simulink model "sf_carcctrl_xpc"  (Simulink 6.0)
settings: Solver=ode4  SolverMode=SingleTasking  StartTime=0.0  StopTime=inf  FixedStep=0.001  RelTol=1e-3  AbsTol=1e-6
PreLoadFcn:
  | load sf_cardat
undefined symbols (not defined in the file or in its folder): converter_data, downtab, emap, Iei, uptab
libraries: xpclib x3, simulink_extras x1
settings Model: CovMetricSettings=d  Creator=nikita  LastModifiedBy=ekbas  ExtModeTrigMode=oneshot  ExtModeArmWhenConnect=off  BufferReuse=off
settings DataIOCC: LimitDataPoints=off  SaveOutput=off  SaveTime=off  SignalLoggingName=sigsOut
settings OptimizationCC: BlockReduction=off  BooleanDataType=off  InlineInvariantSignals=off  OptimizeBlockIOStorage=off  BufferReuse=off  EnforceIntegerDowncast=off  FoldNonRolledExpr=off  LocalBlockOutputs=off
settings DebuggingCC: CheckExecutionContextPreStartOutputMsg=on  CheckExecutionContextRuntimeOutputMsg=on  SolverPrmCheckMsg=none  IntegerOverflowMsg=none
settings RTWCC: SystemTargetFile=xpctarget.tlc  TemplateMakefile=xpc_default_tmf  ProcessScript=xpctarget_make_rtw_hook
settings xpcTargetCC: TargetFcnLib=ansi_tfl_tmw.mat  GenFloatMathFcnCalls=ANSI_C  ModelReferenceCompliant=off  LifeSpan=inf
settings SFSimCC: SFSimApplyToAllLibs=on  SFSimBuildMode=Incremental

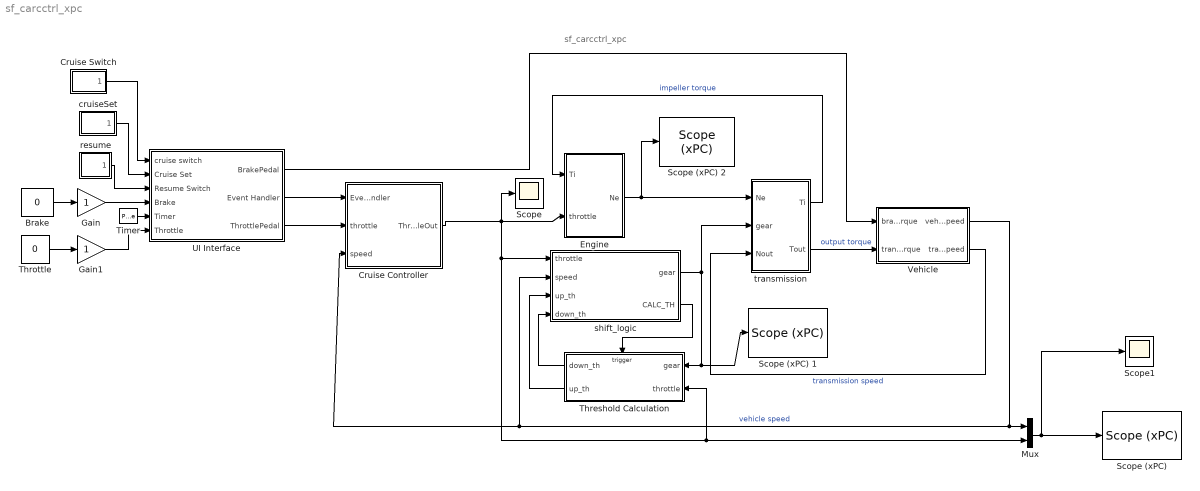
== system sf_carcctrl_xpc ==
  note: sf_carcctrl_xpc
  Brake : Constant  Value=0
  Cruise Controller : Subsystem  PropExecContextAcrossSSBoundary=on
  Cruise Switch : Subsystem  PropExecContextAcrossSSBoundary=on  mask(Manual Switch){sw=1, action=0}
      mask prompts: sw "Current setting:"
      mask help: Output toggles between two inputs by double-clicking on the block.
      mask init:
      | [x,y]=manevent;
      settings: OpenFcn=set_param(gcbh,'action','1');
      mask Help: This block implements a manual switch.
      mask Display: plot(x,y);
  Engine : Subsystem  PropExecContextAcrossSSBoundary=on
  Gain : Gain  SaturateOnIntegerOverflow=on
  Gain1 : Gain  SaturateOnIntegerOverflow=on
  Mux : Mux  Inputs=2
  Scope : Scope
      settings: TimeRange=10  YMin=-1  YMax=1
  "Scope (xPC) " : xpclib/Misc./Scope (xPC)   scopeno=1  scopetype=Target  autostart=on  viewmode=Graphical rolling  formatstr='%15.6f'  grid=on  ylimits=[0,160]  nosamples=1000  noprepostsamples=0  interleave=50  triggermode=FreeRun  triggersignal=1  triggerlevel=0.0  triggerslope=Either  triggerscope=1  triggersample=0  filename=data.dat  mode=Lazy  writesize=512  autorestart=off
  Scope (xPC) 1 : xpclib/Misc./Scope (xPC)   scopeno=3  scopetype=Target  autostart=on  viewmode=Numerical  formatstr='%15.6f'  grid=on  ylimits=[0,180]  nosamples=50  noprepostsamples=0  interleave=1  triggermode=FreeRun  triggersignal=1  triggerlevel=0.0  triggerslope=Either  triggerscope=1  triggersample=0  filename=data.dat  mode=Lazy  writesize=512  autorestart=off
  Scope (xPC) 2 : xpclib/Misc./Scope (xPC)   scopeno=2  scopetype=Target  autostart=on  viewmode=Graphical rolling  formatstr='%15.6f'  grid=on  ylimits=[0,6000]  nosamples=1000  noprepostsamples=0  interleave=50  triggermode=FreeRun  triggersignal=1  triggerlevel=0.0  triggerslope=Either  triggerscope=1  triggersample=0  filename=data.dat  mode=Lazy  writesize=512  autorestart=off
  Scope1 : Scope
      settings: TimeRange=10  YMin=0  YMax=5.5  SaveName=ScopeData2
  Threshold Calculation : Subsystem  Orientation=left  TreatAsAtomicUnit=on  PropExecContextAcrossSSBoundary=on
  Throttle : Constant  Value=0
  Timer : DiscretePulseGenerator  PulseType=Time based  Period=0.05  PulseWidth=50
  UI Interface : Subsystem  PropExecContextAcrossSSBoundary=on
  Vehicle : Subsystem  PropExecContextAcrossSSBoundary=on  mask(vehicle model){@1=vehicledata(1), @2=vehicledata(2), @3=vehicledata(3), @4=vehicledata(4), @5=vehicledata(5), @6=vehicledata(6)/vehicledata(4)*vehicledata(1)}
      mask prompts: @1 "final drive ratio"; @2 "drag friction at wheels"; @3 "aerodynamic drag"; @4 "wheel radius"; @5 "vehicle inertia"; @6 "initial transmission output speed"
      mask help: vehicle dynamics: torque input from trans., outputs are input speed (transmission output) and vehicle speed
      mask init:
      | Rfd = @1; rload0 = @2; rload2 = @3; Rw = @4; Iv = @5; N20 = @6;
      mask Display: plot([cos(pi*[0:5:360]/180) + 6], [sin(pi*[0:5:360]/180) + 1.5],[cos(pi*[0:5:360]/180) + 1], [sin(pi*[0:5:360]/180) + 4], [10 7.5 6.75], [3.5 1 1.5], [10 9.75 7.5 6.25 3 1.5 4 5 7.5], [3.5 4.75 5.5 7 8 7 6 4 5.5], [6.5 4], [7 6], [5.25 2], [2 4], [7.5 1 0], [2.5 6 6.5], [7.5 7.25 9.75], [1 2.25 4.75], [2.75 2 0 0 0.25], [7.5 8 6.5 5.25 5], [1.5 0.5], [6.75 6.25])
  cruiseSet : Subsystem  PropExecContextAcrossSSBoundary=on  mask(Manual Switch){sw=1, action=0}
      mask prompts: sw "Current setting:"
      mask help: Output toggles between two inputs by double-clicking on the block.
      mask init:
      | [x,y]=manevent;
      settings: OpenFcn=set_param(gcbh,'action','1');
      mask Help: This block implements a manual switch.
      mask Display: plot(x,y);
  resume : Subsystem  PropExecContextAcrossSSBoundary=on  mask(Manual Switch){sw=0, action=0}
      mask prompts: sw "Current setting:"
      mask help: Output toggles between two inputs by double-clicking on the block.
      mask init:
      | [x,y]=manevent;
      settings: OpenFcn=set_param(gcbh,'action','1');
      mask Help: This block implements a manual switch.
      mask Display: plot(x,y);
  shift_logic : Stateflow chart  PropExecContextAcrossSSBoundary=on
  transmission : Subsystem  PropExecContextAcrossSSBoundary=on
  wires:
  transmission/1(Ti) -> Engine/1(Ti)  "impeller torque"
  Engine/1(Ne) -> transmission/1(Ne), Scope (xPC) 2/1
  transmission/2(Tout) -> Vehicle/2(transmission output torque)  "output torque"
  Vehicle/2(transmission output speed) -> transmission/3(Nout)  "transmission speed"
  Threshold Calculation/1(down_th) -> shift_logic/4(down_th)
  Threshold Calculation/2(up_th) -> shift_logic/3(up_th)
  shift_logic/1(gear) -> transmission/2(gear), Threshold Calculation/1(gear), Scope (xPC) 1/1
  shift_logic/2(CALC_TH) -> Threshold Calculation/Trigger
  Vehicle/1(vehicle speed) -> Mux/1, shift_logic/2(speed), Cruise Controller/3(speed)  "vehicle speed"
  Mux/1 -> "Scope (xPC) "/1, Scope1/1
  Cruise Controller/1(ThrottleOut) -> shift_logic/1(throttle), Mux/2, Threshold Calculation/2(throttle), Engine/2(throttle), Scope/1
  Throttle/1 -> Gain1/1
  Timer/1 -> UI Interface/5(Timer)
  cruiseSet/1(Output) -> UI Interface/2(Cruise Set)
  resume/1(Output) -> UI Interface/3(Resume Switch)
  Cruise Switch/1(Output) -> UI Interface/1(cruise switch)
  Brake/1 -> Gain/1
  UI Interface/2(Event Handler) -> Cruise Controller/1(Event Handler)
  UI Interface/3(ThrottlePedal) -> Cruise Controller/2(throttle)
  UI Interface/1(BrakePedal) -> Vehicle/1(brake torque)
  Gain/1 -> UI Interface/4(Brake)
  Gain1/1 -> UI Interface/6(Throttle)

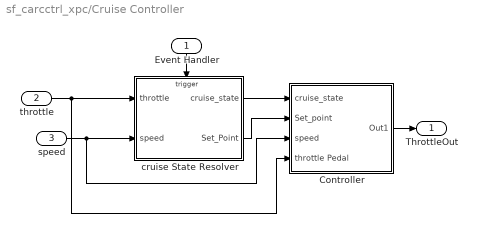
== system sf_carcctrl_xpc/Cruise Controller ==
  Event Handler : Inport  Orientation=down  LatchInput=off
  throttle : Inport  Port=2  LatchInput=off
  speed : Inport  Port=3  LatchInput=off
  Controller : Subsystem  PropExecContextAcrossSSBoundary=on
  cruise State Resolver : Stateflow chart  TreatAsAtomicUnit=on  PropExecContextAcrossSSBoundary=on
  ThrottleOut : Outport
  wires:
  Controller/1(Out1) -> ThrottleOut/1
  Event Handler/1 -> cruise State Resolver/Trigger
  speed/1 -> Controller/3(speed), cruise State Resolver/2(speed)
  throttle/1 -> Controller/4(throttle Pedal), cruise State Resolver/1(throttle)
  cruise State Resolver/2(Set_Point) -> Controller/2(Set_point)
  cruise State Resolver/1(cruise_state) -> Controller/1(cruise_state)

== system sf_carcctrl_xpc/Cruise Switch ==
  Constant : Constant
  Output : Outport
  wires:
  Constant/1 -> Output/1

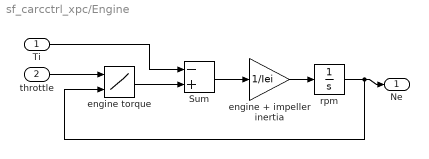
== system sf_carcctrl_xpc/Engine ==
  Ti : Inport  LatchInput=off
  throttle : Inport  Port=2  LatchInput=off
  Sum : Sum  Inputs=-+  SaturateOnIntegerOverflow=on  InputSameDT=on
  engine torque : Lookup2D  DialogController=Simulink.DDGSource  RowIndex=thvec  ColumnIndex=nevec  OutputValues=emap  SaturateOnIntegerOverflow=on  InputSameDT=on
  engine + impeller inertia : Gain  Gain=1/Iei  SaturateOnIntegerOverflow=on
  rpm : Integrator  InitialCondition=1000  LimitOutput=on  UpperSaturationLimit=6000  LowerSaturationLimit=600
  Ne : Outport  InitialOutput=0
  wires:
  Ti/1 -> Sum/1
  throttle/1 -> engine torque/1
  rpm/1 -> engine torque/2, Ne/1
  Sum/1 -> engine + impeller inertia/1
  engine + impeller inertia/1 -> rpm/1
  engine torque/1 -> Sum/2

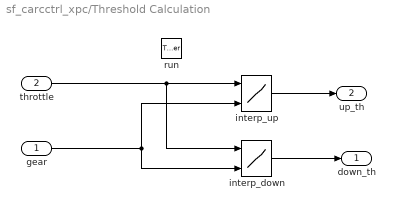
== system sf_carcctrl_xpc/Threshold Calculation ==
  gear : Inport  LatchInput=off
  throttle : Inport  Port=2  LatchInput=off
  run : TriggerPort  TriggerType=function-call  StatesWhenEnabling=reset
  interp_down : Lookup2D  DialogController=Simulink.DDGSource  RowIndex=downth  ColumnIndex=[1:4]  OutputValues=downtab  SaturateOnIntegerOverflow=on  InputSameDT=on
  interp_up : Lookup2D  DialogController=Simulink.DDGSource  RowIndex=upth  ColumnIndex=[1:4]  OutputValues=uptab  SaturateOnIntegerOverflow=on  InputSameDT=on
  down_th : Outport
  up_th : Outport  Port=2
  wires:
  interp_up/1 -> up_th/1
  interp_down/1 -> down_th/1
  throttle/1 -> interp_up/1, interp_down/1
  gear/1 -> interp_up/2, interp_down/2

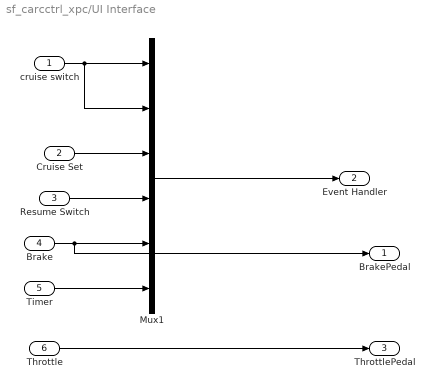
== system sf_carcctrl_xpc/UI Interface ==
  cruise switch : Inport  LatchInput=off
  Cruise Set : Inport  Port=2  LatchInput=off
  Resume Switch : Inport  Port=3  LatchInput=off
  Brake : Inport  Port=4  LatchInput=off
  Timer : Inport  Port=5  LatchInput=off
  Throttle : Inport  Port=6  LatchInput=off
  Mux1 : Mux  Inputs=6
  BrakePedal : Outport
  Event Handler : Outport  Port=2
  ThrottlePedal : Outport  Port=3
  wires:
  Throttle/1 -> ThrottlePedal/1
  Timer/1 -> Mux1/6
  Resume Switch/1 -> Mux1/4
  Cruise Set/1 -> Mux1/3
  cruise switch/1 -> Mux1/1, Mux1/2
  Mux1/1 -> Event Handler/1
  Brake/1 -> BrakePedal/1, Mux1/5

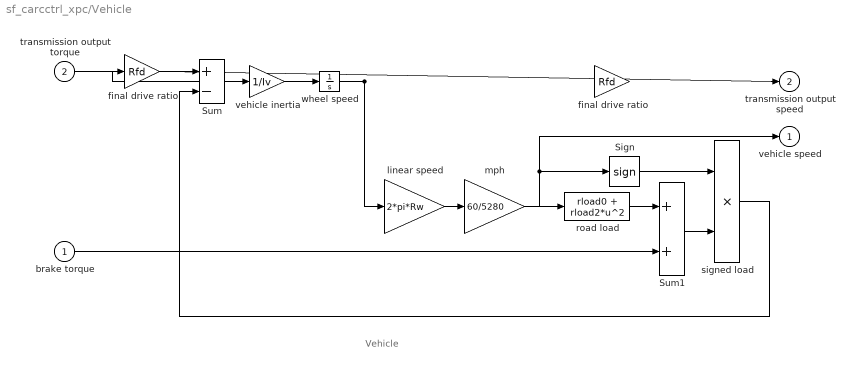
== system sf_carcctrl_xpc/Vehicle ==
  note: Vehicle
  brake torque : Inport  LatchInput=off
  transmission output torque : Inport  Port=2  LatchInput=off
  Sign : Signum
  Sum : Sum  Inputs=+-  SaturateOnIntegerOverflow=on  InputSameDT=on
  Sum1 : Sum  SaturateOnIntegerOverflow=on  InputSameDT=on
  final drive ratio : Gain  Gain=Rfd  SaturateOnIntegerOverflow=on
  final drive ratio : Gain  Gain=Rfd  SaturateOnIntegerOverflow=on
  linear speed : Gain  Gain=2*pi*Rw  SaturateOnIntegerOverflow=on
  mph : Gain  Gain=60/5280  SaturateOnIntegerOverflow=on
  road load : Fcn  Expr=rload0 + rload2*u^2
  signed load : Product  SaturateOnIntegerOverflow=on  InputSameDT=on
  vehicle inertia : Gain  Gain=1/Iv  SaturateOnIntegerOverflow=on
  wheel speed : Integrator  InitialCondition=N20/Rfd
  vehicle speed : Outport  InitialOutput=0
  transmission output speed : Outport  Port=2  InitialOutput=0
  wires:
  final drive ratio/1 -> transmission output speed/1
  brake torque/1 -> Sum1/2
  Sum1/1 -> signed load/2
  road load/1 -> Sum1/1
  Sign/1 -> signed load/1
  signed load/1 -> Sum/2
  transmission output torque/1 -> final drive ratio/1
  vehicle inertia/1 -> wheel speed/1
  Sum/1 -> vehicle inertia/1
  mph/1 -> vehicle speed/1, Sign/1, road load/1
  linear speed/1 -> mph/1
  wheel speed/1 -> linear speed/1, final drive ratio/1
  final drive ratio/1 -> Sum/1

== system sf_carcctrl_xpc/cruiseSet ==
  Constant : Constant
  Output : Outport
  wires:
  Constant/1 -> Output/1

== system sf_carcctrl_xpc/resume ==
  Constant : Constant  Value=0
  Output : Outport
  wires:
  Constant/1 -> Output/1

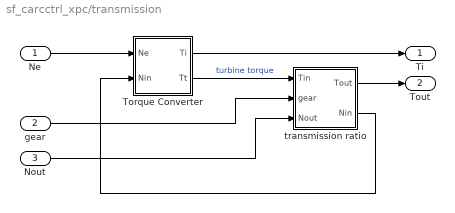
== system sf_carcctrl_xpc/transmission ==
  Ne : Inport  LatchInput=off
  gear : Inport  Port=2  LatchInput=off
  Nout : Inport  Port=3  LatchInput=off
  Torque Converter : Subsystem  PropExecContextAcrossSSBoundary=on  mask(torque converter){speedratio=converter_data(:,1), Kfactor=converter_data(:,2), Torkratio=converter_data(:,3)}
      mask prompts: speedratio "speed ratio"; Kfactor "K factor"; Torkratio "torque ratio"
      mask help: torque converter
      mask Help: Torque converter input and output torques are computed as a function of the input and output speeds
      mask Display: plot([cos([90:10:450]*pi/180),.63*cos([90:10:450]*pi/180),.63*cos([90:10:240]*pi/180),cos([240:10:300]*pi/180),.63*cos([300]*pi/180)],[sin([90:10:450]*pi/180),.63*sin([90:10:450]*pi/180)+.1,.63*sin([90:10:240]*pi/180)+.1,sin([240:10:300]*pi/180),.63*sin([300]*pi/180)+.1])
  transmission ratio : Subsystem  PropExecContextAcrossSSBoundary=on
  Ti : Outport  InitialOutput=0
  Tout : Outport  Port=2  InitialOutput=0
  wires:
  transmission ratio/1(Tout) -> Tout/1
  Torque Converter/1(Ti) -> Ti/1
  Nout/1 -> transmission ratio/3(Nout)
  gear/1 -> transmission ratio/2(gear)
  Ne/1 -> Torque Converter/1(Ne)
  transmission ratio/2(Nin) -> Torque Converter/2(Nin)
  Torque Converter/2(Tt) -> transmission ratio/1(Tin)  "turbine torque"

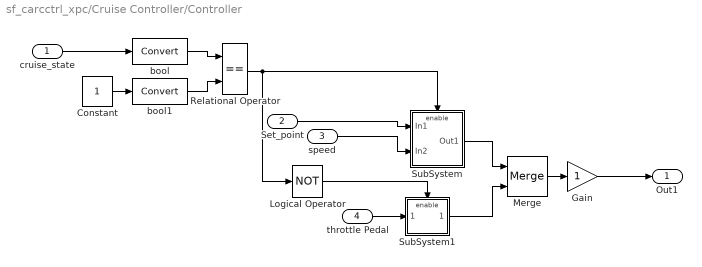
== system sf_carcctrl_xpc/Cruise Controller/Controller ==
  cruise_state : Inport  LatchInput=off
  Set_point : Inport  Port=2  LatchInput=off
  speed : Inport  Port=3  LatchInput=off
  throttle Pedal : Inport  Port=4  LatchInput=off
  Constant : Constant
  Gain : Gain  SaturateOnIntegerOverflow=on
  Logical Operator : Logic  Operator=NOT
  Merge : Merge
  Relational Operator : RelationalOperator  Operator===  InputSameDT=on
  SubSystem : Subsystem  TreatAsAtomicUnit=on  PropExecContextAcrossSSBoundary=on
  SubSystem1 : Subsystem  TreatAsAtomicUnit=on  PropExecContextAcrossSSBoundary=on
  bool : DataTypeConversion  OutDataTypeMode=boolean  SaturateOnIntegerOverflow=on  RndMeth=Zero
  bool1 : DataTypeConversion  OutDataTypeMode=boolean  SaturateOnIntegerOverflow=on  RndMeth=Zero
  Out1 : Outport  InitialOutput=0
  wires:
  Gain/1 -> Out1/1
  Merge/1 -> Gain/1
  SubSystem1/1(Out1) -> Merge/2
  SubSystem/1(Out1) -> Merge/1
  Logical Operator/1 -> SubSystem1/Enable
  Relational Operator/1 -> Logical Operator/1, SubSystem/Enable
  bool1/1 -> Relational Operator/2
  bool/1 -> Relational Operator/1
  throttle Pedal/1 -> SubSystem1/1(In1)
  Set_point/1 -> SubSystem/1(In1)
  Constant/1 -> bool1/1
  cruise_state/1 -> bool/1
  speed/1 -> SubSystem/2(In2)

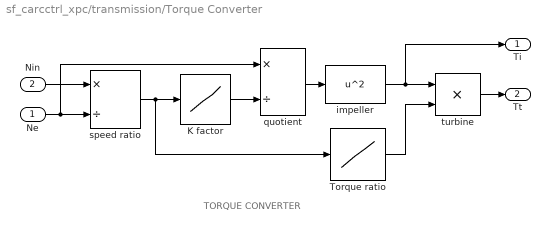
== system sf_carcctrl_xpc/transmission/Torque Converter ==
  note: TORQUE CONVERTER
  Ne : Inport  LatchInput=off
  Nin : Inport  Port=2  LatchInput=off
  K factor : Lookup  DialogController=Simulink.DDGSource  InputValues=speedratio  OutputValues=Kfactor  SaturateOnIntegerOverflow=on
  Torque ratio : Lookup  DialogController=Simulink.DDGSource  InputValues=speedratio  OutputValues=Torkratio  SaturateOnIntegerOverflow=on
  impeller : Fcn  Expr=u^2
  quotient : Product  Inputs=*/  SaturateOnIntegerOverflow=on  InputSameDT=on
  speed ratio : Product  Inputs=*/  SaturateOnIntegerOverflow=on  InputSameDT=on
  turbine : Product  SaturateOnIntegerOverflow=on  InputSameDT=on
  Ti : Outport  InitialOutput=0
  Tt : Outport  Port=2  InitialOutput=0
  wires:
  Torque ratio/1 -> turbine/2
  quotient/1 -> impeller/1
  K factor/1 -> quotient/2
  speed ratio/1 -> Torque ratio/1, K factor/1
  impeller/1 -> turbine/1, Ti/1
  turbine/1 -> Tt/1
  Ne/1 -> speed ratio/2, quotient/1
  Nin/1 -> speed ratio/1

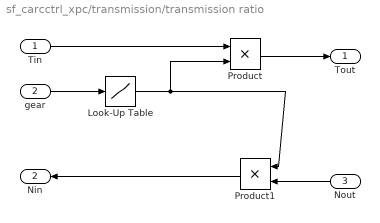
== system sf_carcctrl_xpc/transmission/transmission ratio ==
  Tin : Inport  LatchInput=off
  gear : Inport  Port=2  LatchInput=off
  Nout : Inport  Orientation=left  Port=3  LatchInput=off
  Look-Up Table : Lookup  DialogController=Simulink.DDGSource  InputValues=[1 2 3 4]  OutputValues=[2.393 1.450 1.000 0.677]  SaturateOnIntegerOverflow=on
  Product : Product  SaturateOnIntegerOverflow=on  InputSameDT=on
  Product1 : Product  Orientation=left  SaturateOnIntegerOverflow=on  InputSameDT=on
  Tout : Outport  InitialOutput=0
  Nin : Outport  Orientation=left  Port=2  InitialOutput=0
  wires:
  Look-Up Table/1 -> Product1/1, Product/2
  Nout/1 -> Product1/2
  Product1/1 -> Nin/1
  Product/1 -> Tout/1
  Tin/1 -> Product/1
  gear/1 -> Look-Up Table/1

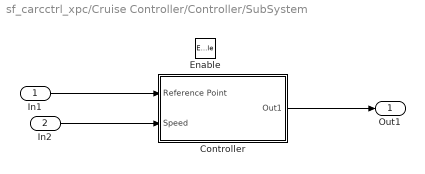
== system sf_carcctrl_xpc/Cruise Controller/Controller/SubSystem ==
  In1 : Inport  LatchInput=off
  In2 : Inport  Port=2  LatchInput=off
  Enable : EnablePort
  Controller : Subsystem  PropExecContextAcrossSSBoundary=on
  Out1 : Outport
  wires:
  In1/1 -> Controller/1(Reference Point)
  In2/1 -> Controller/2(Speed)
  Controller/1(Out1) -> Out1/1

== system sf_carcctrl_xpc/Cruise Controller/Controller/SubSystem1 ==
  In1 : Inport  LatchInput=off
  Enable : EnablePort
  Out1 : Outport
  wires:
  In1/1 -> Out1/1

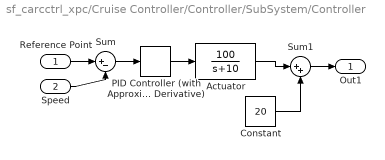
== system sf_carcctrl_xpc/Cruise Controller/Controller/SubSystem/Controller ==
  Reference Point : Inport  LatchInput=off
  Speed : Inport  Port=2  LatchInput=off
  Actuator : TransferFcn  Numerator=[100]  Denominator=[1 10]
  Constant : Constant  Value=20
  PID Controller (with Approximate Derivative) : simulink_extras/Additional Linear/PID Controller (with Approximate Derivative)  P=1.5  I=0  D=0  N=100
  Sum : Sum  Inputs=|+-  SaturateOnIntegerOverflow=on  InputSameDT=on
  Sum1 : Sum  Inputs=|++  SaturateOnIntegerOverflow=on  InputSameDT=on
  Out1 : Outport
  wires:
  Speed/1 -> Sum/2
  Sum1/1 -> Out1/1
  Reference Point/1 -> Sum/1
  Constant/1 -> Sum1/2
  Actuator/1 -> Sum1/1
  PID Controller (with Approximate Derivative)/1 -> Actuator/1
  Sum/1 -> PID Controller (with Approximate Derivative)/1

== stateflow chart shift_logic ==
  settings: updateMethod=DISCRETE  sampleTime=0.001
  state gear_state [parallel]
    state fourth
      entry: gear = 4;
    state second
      entry: gear = 2;
    state third
      entry: gear = 3;
    state first
      entry: gear = 1;
    third -> fourth : UP
    second -> third : UP
    first -> second : UP
    (default) -> first
    fourth -> third : DOWN
    third -> second : DOWN
    second -> first : DOWN
  state selection_state [parallel]
    during: CALC_TH;
    state downshifting
    state upshifting
    state steady_state
    (default) -> steady_state
    steady_state -> upshifting : [speed > up_th]
    steady_state -> downshifting : [speed < down_th]
    upshifting -> steady_state : [speed < up_th]
    downshifting -> steady_state : [speed > down_th]
    downshifting -> steady_state : after(TWAIT,tick)
        | [speed <= down_th]
        | {gear_state.DOWN}
    upshifting -> steady_state : after(TWAIT,tick)
        | [speed >= up_th]
        | {gear_state.UP}
  data: throttle input double; speed input double; gear output uint8 [1..4]; TWAIT parameter uint8; up_th input double; down_th input double
  data throttle settings: units=double
  data speed settings: units=double
  data gear settings: units=int
  events: DOWN local EITHER_EDGE_EVENT; UP local EITHER_EDGE_EVENT; CALC_TH output FUNCTION_CALL_EVENT

== stateflow chart Cruise Controller/cruise State Resolver ==
  state cruiseoff
    cruise_state=0;
  state cruiseon
    cruise_state=0;
  state KeepSpeed
    cruise_state=1;
  state Suspend
    cruise_state=0;
  state increase_decrease
    cruise_state=0;
  (default) -> cruiseoff
  cruiseoff -> cruiseon : cruise_on[speed >45]
  cruiseon -> cruiseoff : cruise_off
  cruiseon -> KeepSpeed : cruise_set/Set_Point=speed;throtval=throttle;
  increase_decrease -> (junction 42) : cruise_off
  KeepSpeed -> Suspend : brake
  Suspend -> KeepSpeed : resume
  Suspend -> cruiseoff : cruise_off
  increase_decrease -> KeepSpeed : timer[throttle==throtval]
  KeepSpeed -> increase_decrease : timer[throttle>throtval || throttle < throtval]
  increase_decrease -> KeepSpeed : cruise_set/Set_Point=speed;throtval=throttle;
  KeepSpeed -> (junction 42) : cruise_off
  (junction 42) -> cruiseoff
  increase_decrease -> KeepSpeed : resume
  data: throttle input double; speed input double; cruise_state output double; Set_Point output double; throtval local double
  events: cruise_on input RISING_EDGE_EVENT; cruise_off input FALLING_EDGE_EVENT; cruise_set input EITHER_EDGE_EVENT; resume input EITHER_EDGE_EVENT; brake input RISING_EDGE_EVENT; timer input EITHER_EDGE_EVENT
